simulink model "LOES"  (R2025b)
settings: Solver=VariableStepAuto  StartTime=0.0  StopTime=10.0  RelTol=1e-3
undefined symbols (not defined in the file): ActTC
libraries: simulink_extras x6, aerolibactuator x1
settings Model: Creator=Willi  LastModifiedBy=seans

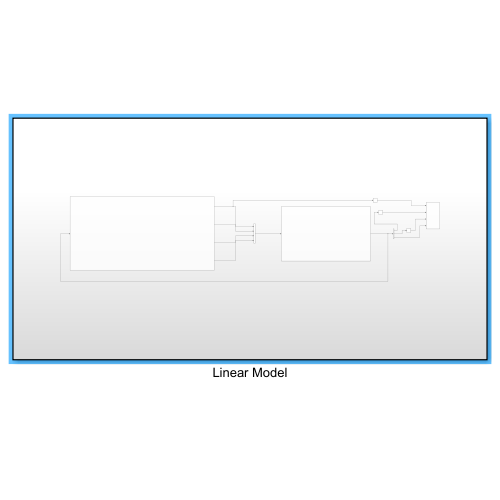
[thumbnail: Simulink's stored preview of the top-level diagram]
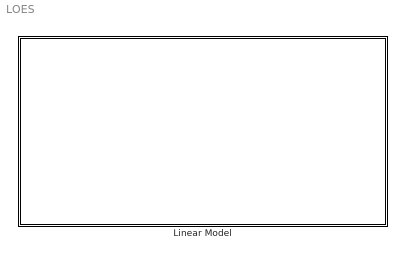
== system LOES ==
  Linear Model : Subsystem

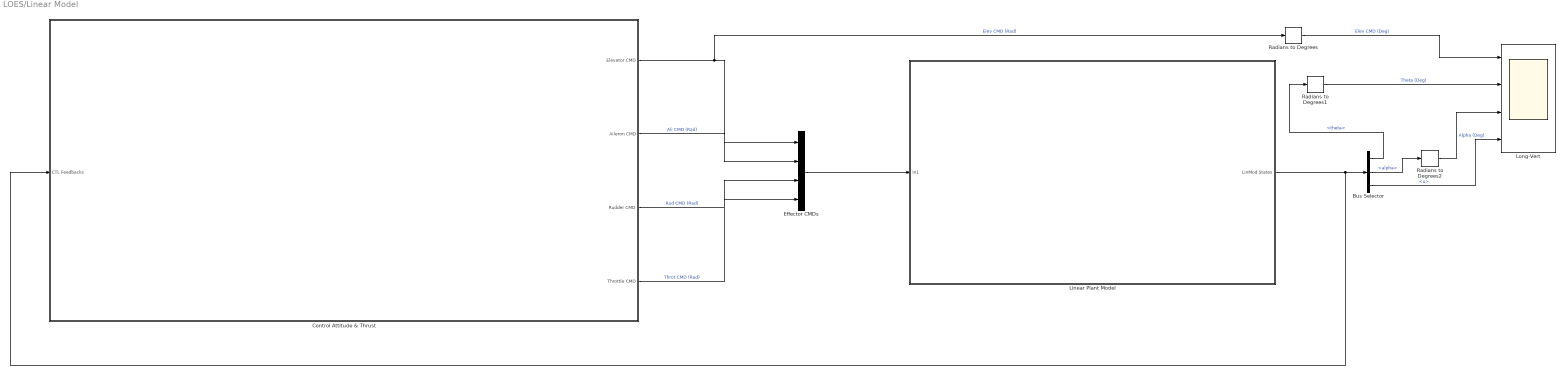
== system LOES/Linear Model ==
  Bus Selector : BusSelector  OutputSignals=theta,alpha,u
  Control Attitude & Thrust : Subsystem
  Effector CMDs : BusCreator  Inputs=4
  Linear Plant Model : Subsystem
  Long-Vert : Scope  NumInputPorts=4
      settings: ActiveDisplayYMinimum=0.019193881170770477  ActiveDisplayYMaximum=5.5534229020921364  DataLoggingVariableName=ScopeData12
  Radians to Degrees : simulink_extras/Transformations/Radians to Degrees
  Radians to Degrees1 : simulink_extras/Transformations/Radians to Degrees
  Radians to Degrees2 : simulink_extras/Transformations/Radians to Degrees
  wires:
  Control Attitude & Thrust/4(Throttle CMD) -> Effector CMDs/4  "Throt CMD (Rad)"
  Effector CMDs/1 -> Linear Plant Model/1(In1)
  Control Attitude & Thrust/2(Aileron CMD) -> Effector CMDs/2  "Ali CMD (Rad)"
  Control Attitude & Thrust/3(Rudder CMD) -> Effector CMDs/3  "Rud CMD (Rad)"
  Control Attitude & Thrust/1(Elevator CMD) -> Radians to Degrees/1, Effector CMDs/1  "Elev CMD (Rad)"
  Linear Plant Model/1(LinMod States) -> Control Attitude & Thrust/1(CTL Feedbacks), Bus Selector/1
  Radians to Degrees/1 -> Long-Vert/1  "Elev CMD (Deg)"
  Bus Selector/1 -> Radians to Degrees1/1  "<theta>"
  Radians to Degrees1/1 -> Long-Vert/2  "Theta (Deg)"
  Bus Selector/2 -> Radians to Degrees2/1  "<alpha>"
  Radians to Degrees2/1 -> Long-Vert/3  "Alpha (Deg)"
  Bus Selector/3 -> Long-Vert/4  "<u>"

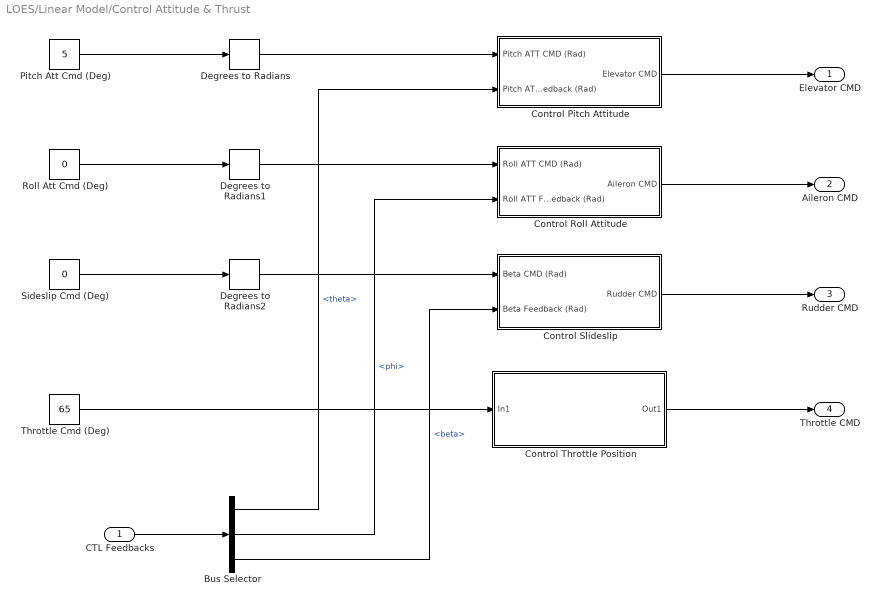
== system LOES/Linear Model/Control Attitude & Thrust ==
  CTL Feedbacks : Inport
  Bus Selector : BusSelector  OutputSignals=theta,phi,beta
  Control Pitch Attitude : Subsystem
  Control Roll Attitude : Subsystem
  Control Slideslip : Subsystem
  Control Throttle Position : Subsystem
  Degrees to Radians : simulink_extras/Transformations/Degrees to Radians
  Degrees to Radians1 : simulink_extras/Transformations/Degrees to Radians
  Degrees to Radians2 : simulink_extras/Transformations/Degrees to Radians
  Pitch Att Cmd (Deg) : Constant  Value=5
  Roll Att Cmd (Deg) : Constant  Value=0
  Sideslip Cmd (Deg) : Constant  Value=0
  Throttle Cmd (Deg) : Constant  Value=65
  Elevator CMD : Outport
  Aileron CMD : Outport  Port=2
  Rudder CMD : Outport  Port=3
  Throttle CMD : Outport  Port=4
  wires:
  Control Throttle Position/1(Out1) -> Throttle CMD/1
  Control Pitch Attitude/1(Elevator CMD) -> Elevator CMD/1
  Throttle Cmd (Deg)/1 -> Control Throttle Position/1(In1)
  Degrees to Radians1/1 -> Control Roll Attitude/1(Roll ATT CMD (Rad))
  Degrees to Radians2/1 -> Control Slideslip/1(Beta CMD (Rad))
  Sideslip Cmd (Deg)/1 -> Degrees to Radians2/1
  Roll Att Cmd (Deg)/1 -> Degrees to Radians1/1
  Pitch Att Cmd (Deg)/1 -> Degrees to Radians/1
  Degrees to Radians/1 -> Control Pitch Attitude/1(Pitch ATT CMD (Rad))
  CTL Feedbacks/1 -> Bus Selector/1
  Bus Selector/1 -> Control Pitch Attitude/2(Pitch ATT Feedback (Rad))  "<theta>"
  Bus Selector/2 -> Control Roll Attitude/2(Roll ATT Feedback (Rad))  "<phi>"
  Bus Selector/3 -> Control Slideslip/2(Beta Feedback (Rad))  "<beta>"
  Control Roll Attitude/1(Aileron CMD) -> Aileron CMD/1
  Control Slideslip/1(Rudder CMD) -> Rudder CMD/1

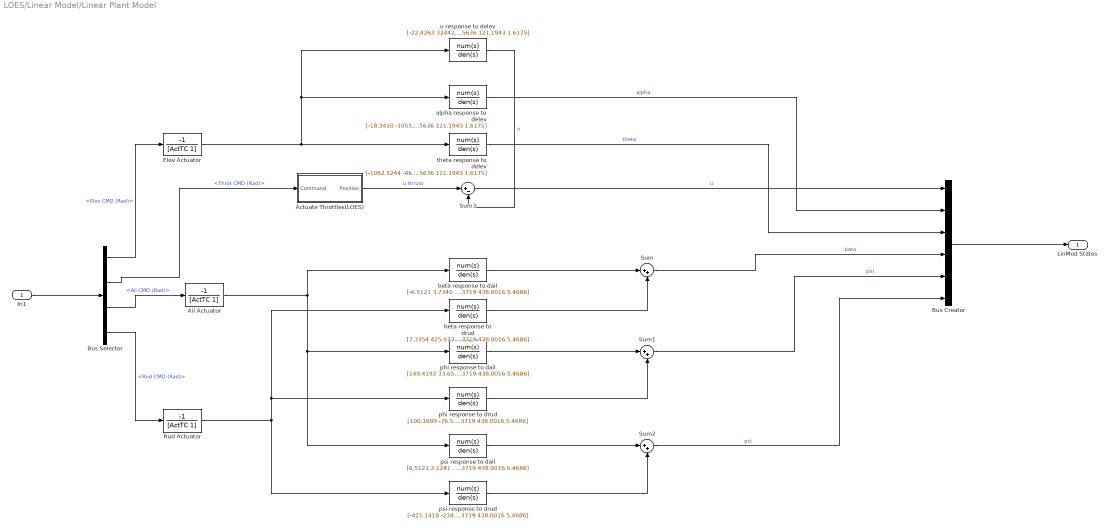
== system LOES/Linear Model/Linear Plant Model ==
  In1 : Inport
  " u response to delev" : TransferFcn  Numerator=[-22.4263 32442.6029 12108.4240]  Denominator=[878.5677 888.9681 1599.5636 121.1943 1.6175]
  Actuate Throttles(LOES) : Subsystem
  Ail Actuator : TransferFcn  Numerator=[-1]  Denominator=[ActTC 1]
  Bus Creator : BusCreator  Inputs=6
  Bus Selector : BusSelector  OutputSignals=Elev CMD (Rad),Throt CMD (Rad),Ali CMD (Rad),Rud CMD (Rad)
  Elev Actuator : TransferFcn  Numerator=[-1]  Denominator=[ActTC 1]
  Rud Actuator : TransferFcn  Numerator=[-1]  Denominator=[ActTC 1]
  Sum : Sum  Inputs=|++
  Sum1 : Sum  Inputs=|++
  Sum2 : Sum  Inputs=|++
  Sum3 : Sum  Inputs=|+-
  alpha response to delev : TransferFcn  Numerator=[-18.3410 -1055.6956 -84.9709 -1.9952]  Denominator=[878.5677 888.9681 1599.5636 121.1943 1.6175]
  beta response to dail : TransferFcn  Numerator=[-6.5121 3.7340 .8827]  Denominator=[870.7830 628.6269 791.3719 438.0016 5.4686]
  beta response to drud : TransferFcn  Numerator=[7.3354 425.9739 218.0615 -2.4517]  Denominator=[870.7830 628.6269 791.3719 438.0016 5.4686]
  phi response to dail : TransferFcn  Numerator=[149.4192 33.6557 133.0699]  Denominator=[870.7830 628.6269 791.3719 438.0016 5.4686]
  phi response to drud : TransferFcn  Numerator=[100.1689 -76.5459 -823.1939]  Denominator=[870.7830 628.6269 791.3719 438.0016 5.4686]
  psi response to dail : TransferFcn  Numerator=[6.5121 2.1241 .1082 4.7950]  Denominator=[870.7830 628.6269 791.3719 438.0016 5.4686]
  psi response to drud : TransferFcn  Numerator=[-421.1418 -234.6564 -10.4259 -29.8066]  Denominator=[870.7830 628.6269 791.3719 438.0016 5.4686]
  theta response to delev : TransferFcn  Numerator=[-1062.5244 -468.6144 -31.4031]  Denominator=[878.5677 888.9681 1599.5636 121.1943 1.6175]
  LinMod States : Outport
  wires:
  phi response to drud/1 -> Sum1/2
  beta response to drud/1 -> Sum/2
  Sum1/1 -> Bus Creator/5  "phi"
  phi response to dail/1 -> Sum1/1
  Sum2/1 -> Bus Creator/6  "psi"
  Sum/1 -> Bus Creator/4  "beta"
  beta response to dail/1 -> Sum/1
  theta response to delev/1 -> Bus Creator/3  "theta"
  Bus Creator/1 -> LinMod States/1
  psi response to dail/1 -> Sum2/1
  psi response to drud/1 -> Sum2/2
  alpha response to delev/1 -> Bus Creator/2  "alpha"
  In1/1 -> Bus Selector/1
  " u response to delev"/1 -> Sum3/2  "u"
  Bus Selector/1 -> Elev Actuator/1  "<Elev CMD (Rad)>"
  Bus Selector/4 -> Rud Actuator/1  "<Rud CMD (Rad)>"
  Bus Selector/3 -> Ail Actuator/1  "<Ali CMD (Rad)>"
  Elev Actuator/1 -> alpha response to delev/1, " u response to delev"/1, theta response to delev/1
  Ail Actuator/1 -> beta response to dail/1, psi response to dail/1, phi response to dail/1
  Rud Actuator/1 -> beta response to drud/1, phi response to drud/1, psi response to drud/1
  Bus Selector/2 -> Actuate Throttles(LOES)/1(Command)  "<Throt CMD (Rad)>"
  Actuate Throttles(LOES)/1(Position) -> Sum3/1  "u thrust"
  Sum3/1 -> Bus Creator/1  "u"

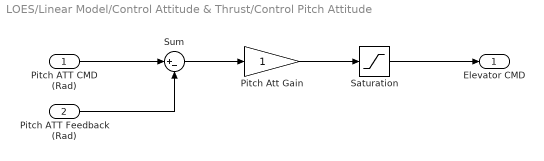
== system LOES/Linear Model/Control Attitude & Thrust/Control Pitch Attitude ==
  Pitch ATT CMD (Rad) : Inport
  Pitch ATT Feedback (Rad) : Inport  Port=2
  Pitch Att Gain : Gain
  Saturation : Saturate  UpperLimit=30  LowerLimit=-30
  Sum : Sum  Inputs=|+-
  Elevator CMD : Outport
  wires:
  Pitch ATT Feedback (Rad)/1 -> Sum/2
  Pitch ATT CMD (Rad)/1 -> Sum/1
  Sum/1 -> Pitch Att Gain/1
  Pitch Att Gain/1 -> Saturation/1
  Saturation/1 -> Elevator CMD/1

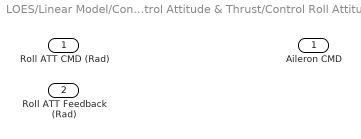
== system LOES/Linear Model/Control Attitude & Thrust/Control Roll Attitude ==
  Roll ATT CMD (Rad) : Inport
  Roll ATT Feedback (Rad) : Inport  Port=2
  Aileron CMD : Outport

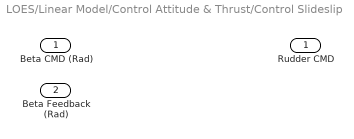
== system LOES/Linear Model/Control Attitude & Thrust/Control Slideslip ==
  Beta CMD (Rad) : Inport
  Beta Feedback (Rad) : Inport  Port=2
  Rudder CMD : Outport

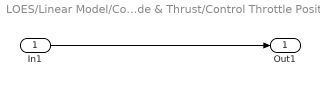
== system LOES/Linear Model/Control Attitude & Thrust/Control Throttle Position ==
  In1 : Inport
  Out1 : Outport
  wires:
  In1/1 -> Out1/1

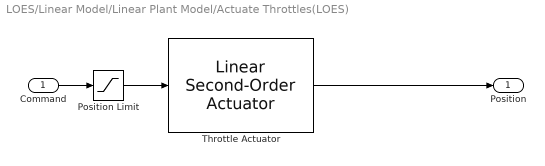
== system LOES/Linear Model/Linear Plant Model/Actuate Throttles(LOES) ==
  Command : Inport
  Position Limit : Saturate  UpperLimit=1  LowerLimit=0
  Throttle Actuator : aerolibactuator/Linear Second-Order Actuator  wn_fin=1  z_fin=1.0  fin_act_0=EngineThrustCMD  fin_act_vel=0
  Position : Outport
  wires:
  Throttle Actuator/1 -> Position/1
  Command/1 -> Position Limit/1
  Position Limit/1 -> Throttle Actuator/1
